simulink model "Loops2"  (Simulink 8.7)
settings: Solver=ode45  StartTime=0.0  StopTime=10.0  RelTol=1e-3
settings Model: Creator=scaife  LastModifiedBy=bourbouh  ExtModeAutoUpdateStatusClock=off
settings DataIOCC: SignalLoggingSaveFormat=ModelDataLogs  SignalLoggingName=sigsOut
settings OptimizationCC: InitFltsAndDblsToZero=on
settings DebuggingCC: SaveWithParameterizedLinksMsg=none  SignalResolutionControl=TryResolveAllWithWarning  MultiTaskDSMMsg=warning  MultiTaskCondExecSysMsg=none
settings HardwareCC: TargetUnknown=on
settings SFSimCC: SimParseCustomCode=off
settings GRTTargetCC: TargetFcnLib=ansi_tfl_tmw.mat  ModelReferenceCompliant=off  ParMdlRefBuildCompliant=off  CompOptLevelCompliant=off  ConcurrentExecutionCompliant=off  GeneratePreprocessorConditionals=Use local settings  CombineOutputUpdateFcns=off  MatFileLogging=off  MATLABClassNameForMDSCustomization=Simulink.SoftwareTarget.TargetSpecificTriggerConfigurationBase  GRTInterface=on

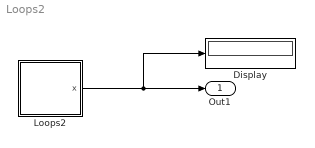
== system Loops2 ==
  Display : Display
  Loops2 : Stateflow chart  TreatAsAtomicUnit=on
  Out1 : Outport
  wires:
  Loops2/1(x) -> Out1/1, Display/1

== stateflow chart Loops2 ==
  state A
  state B
  (default) -> A
  A -> (junction 6) : {x=0}
  (junction 6) -> (junction 6) [order 2] : [x<4]{x+=2}
  (junction 6) -> (junction 6) [order 1] : [x<2]{x++}
  (junction 6) -> B [order 3]
  data: x output int32
